simulink model "Project_Three_1s_Pattern"  (R2020b)
settings: Solver=VariableStepAuto  StartTime=0.0  StopTime=1  RelTol=1e-3
settings Model: Creator=ricar  LastModifiedBy=ricar

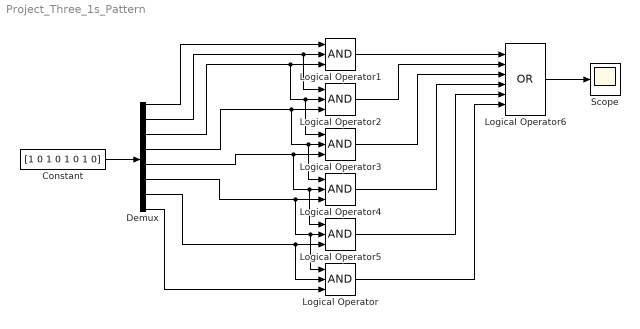
== system Project_Three_1s_Pattern ==
  Constant : Constant  Value=[1 0 1 0 1 0 1 0]
  Demux : Demux  Outputs=8
  Logical Operator{,1..5} (6 alike) : Logic  Inputs=3  IconShape=distinctive  AllPortsSameDT=off  OutDataTypeStr=boolean
  Logical Operator6 : Logic  Operator=OR  Inputs=6  IconShape=distinctive  AllPortsSameDT=off  OutDataTypeStr=boolean
  Scope : Scope
  wires:
  Constant/1 -> Demux/1
  Demux/1 -> Logical Operator1/1
  Demux/2 -> Logical Operator2/1, Logical Operator1/2
  Demux/3 -> Logical Operator3/1, Logical Operator2/2, Logical Operator1/3
  Demux/5 -> Logical Operator5/1, Logical Operator4/2, Logical Operator3/3
  Demux/6 -> Logical Operator/1, Logical Operator5/2, Logical Operator4/3
  Demux/4 -> Logical Operator4/1, Logical Operator3/2, Logical Operator2/3
  Demux/7 -> Logical Operator/2, Logical Operator5/3
  Demux/8 -> Logical Operator/3
  Logical Operator1/1 -> Logical Operator6/1
  Logical Operator2/1 -> Logical Operator6/2
  Logical Operator3/1 -> Logical Operator6/3
  Logical Operator4/1 -> Logical Operator6/4
  Logical Operator5/1 -> Logical Operator6/5
  Logical Operator/1 -> Logical Operator6/6
  Logical Operator6/1 -> Scope/1
